simulink model "main_gilbert_R2022b"  (R2022b)
settings: Solver=VariableStepAuto  StartTime=0.0  StopTime=1  FixedStep=0.01  RelTol=1e-3
libraries: dspsigops x3, commchan3 x2, simulink x2, commsink2 x2, dspvision x2, commblkcod2 x2, commdigbbndpm3 x2, commfilt2 x2, dspstat3 x1, commrandsrc3 x1
settings Model: Creator=avyamalhotra  LastModifiedBy=Tenna Yuan

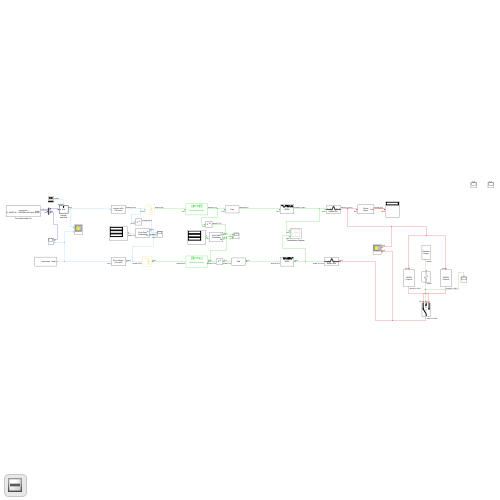
[thumbnail: Simulink's stored preview of the top-level diagram]
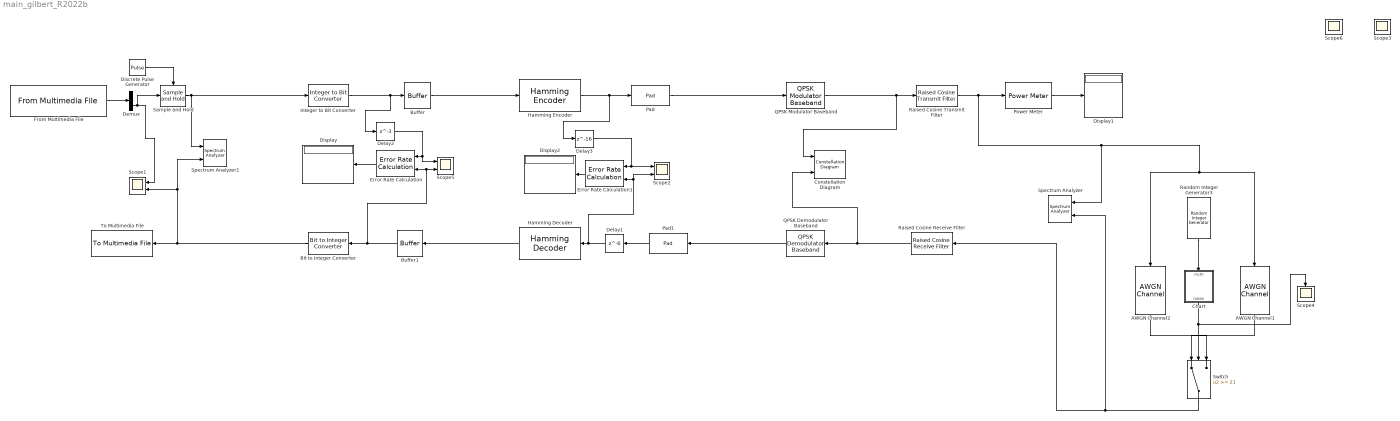
== system main_gilbert_R2022b ==
  AWGN Channel1 : commchan3/AWGN Channel  InputProcessing=Columns as channels (frame based)  noiseMode="Signal to noise ratio  (SNR)"  EbNodB=2  EsNodB=10  SNRdB=21  bitsPerSym=4  Ps=1  Tsym=(9.765625e-08 * 1)  variance=1  seed=67
  AWGN Channel2 : commchan3/AWGN Channel  InputProcessing=Columns as channels (frame based)  noiseMode="Signal to noise ratio  (SNR)"  EbNodB=2  EsNodB=10  SNRdB=9  bitsPerSym=4  Ps=1  Tsym=(9.765625e-08 * 1)  variance=1  seed=67
  Bit to Integer Converter : simulink/Logic and Bit Operations/Bit to Integer Converter  nbits=32  bitOrder=MSB first  signedOutputValues=Signed  outDtype=Inherit via internal rule  outDtypeSigned=int16
  Buffer : Buffer  N=4  OutputFrames=off
  Buffer1 : Buffer  N=32  OutputFrames=off
  Chart : Stateflow chart  TreatAsAtomicUnit=on
  Constellation Diagram : ConstellationDiagram  NumInputPorts=2  WindowPosition=[382.000000,84.000000,600.000000,600.000000,]  ScopeFrameLocation=window  SamplesPerSymbol=100  SymbolsToDisplaySource=Property  SymbolsToDisplay=200  ReferenceConstellation="{[0.70711+0.70711i        -0.70711+0.70711i        -0.70711-0.70711i         0.70711-0.70711i][0.7071+0.7071i          -0.7071+0.7071i          -0.7071-0.7071i            0.707-0.7071i]}"  XLimits=[-1.46,1.46]  YLimits=[-1.38,1.38]  ShowLegend=on
  Delay1 : Delay  DelayLength=6  InitialCondition=0
  Delay2 : Delay  DelayLength=3  InitialCondition=0
  Delay3 : Delay  DelayLength=16  InitialCondition=0
  Demux : Demux  Outputs=2
  Discrete Pulse Generator : DiscretePulseGenerator  SampleTime=1/40000
  Display : Display
  Display1 : Display
  Display2 : Display
  Error Rate Calculation : commsink2/Error Rate Calculation  N=0  st_delay=0  cp_mode=Entire frame  subframe=[]  PMode=Port  WsName=ErrorVec  RsMode2=off  stop=off  numErr=100  maxBits=1e6
  Error Rate Calculation1 : commsink2/Error Rate Calculation  N=0  st_delay=0  cp_mode=Entire frame  subframe=[]  PMode=Port  WsName=ErrorVec  RsMode2=off  stop=off  numErr=100  maxBits=1e6
  From Multimedia File : dspvision/From Multimedia File  inputFilename=D:\Documents\Uni\Year_3\Academics\ELEC_391\ELEC391-Communications-Systems\Simulink component\sound.wav  readRange=[1 Inf]  loop=on  numPlays=1  outputStreams=Audio only  videoDataType=single  audioDataType=int16  inheritSampleTime=on  userDefinedSampleTime=1/30  noAudioOutput=off  isIntensityVideo=off  fourcc=RGB  colorVideoFormat=Separate color signals  outputEOF=off  dataOrg=Column-major  audioFrameSize=1  computeAudioFrameSize=off  outSamplingMode=Sample based
      settings: LibrarySourceBlock=dspsrcs4/From Multimedia File
  Hamming Decoder : commblkcod2/Hamming Decoder  n=7  k=4
  Hamming Encoder : commblkcod2/Hamming Encoder  n=7  k=4
  Integer to Bit Converter : simulink/Logic and Bit Operations/Integer to Bit Converter  nbits=32  signedInputValues=Signed  bitOrder=MSB first  outDtype=double
  Pad : dspsigops/Pad  padAlong=Columns  dimsToPad=1  valSrc=Specify via dialog  padVal=0  spec=Output size  padNumOutRowsSpecMethod=User-specified  numOutRows=8  padNumOutColsSpecMethod=User-specified  numOutCols=7  isVarDimsMode=off  padBeginning=0  padEnd=0  outSizeMode=User-specified  outSize=1  padSigAt=End  trunc_flag=None  roundingMode=Floor  overflowMode=off  truncOrWrapMode=Truncate  wrap_flag=None
  Pad1 : dspsigops/Pad  padAlong=Columns  dimsToPad=1  valSrc=Specify via dialog  padVal=0  spec=Output size  padNumOutRowsSpecMethod=User-specified  numOutRows=7  padNumOutColsSpecMethod=User-specified  numOutCols=1  isVarDimsMode=off  padBeginning=0  padEnd=0  outSizeMode=User-specified  outSize=1  padSigAt=End  trunc_flag=None  roundingMode=Floor  overflowMode=off  truncOrWrapMode=Truncate  wrap_flag=None
  Power Meter : dspstat3/Power Meter  Measurement=Average power  ReferenceLoad=1  OutputPowerUnits=Watts  WindowLength=256  OverlapLength=255  AllowArbitraryInputLength=on  ComputeCCDF=off  PowerRange=50  PowerResolution=0.1  CCDFOutput=Relative power (dB above average power)  ProbabilityVector=[ 10; 1; 0.1; 0.01; 0.001; 0.0001 ]  RelativePowerVector=[ 0; 3; 6; 9; 12 ]  ResetPort=off  SimulateUsing=Code generation
      settings: LibrarySourceBlock=commutil2/Power Meter
  QPSK Demodulator Baseband : commdigbbndpm3/QPSK Demodulator Baseband  OutType=Bit  DecType=Hard decision  VarSource=Dialog  Variance=1  Dec=Gray  Ph=pi/4  outDtype1=Inherit via internal rule  outDtype2=Inherit via internal rule  derotateFactorWordLen=16  derotateFactorDataTypeStr=Inherit: Same word length as input  derotateFactorLastDataTypeStr=Inherit: Same word length as input
  QPSK Modulator Baseband : commdigbbndpm3/QPSK Modulator Baseband  InType=Bit  Enc=Gray  Ph=pi/4  outDtype=double  outWordLen=16  outUDDataType=sfix(16)  outFracLenMode=Best precision  outFracLen=15  outDataTypeStr=double  outLastDataTypeStr=double
  Raised Cosine Receive Filter : commfilt2/Raised Cosine Receive Filter  filtType=Square root  R=0.001  filtSpan=10  N=8  downFactor=8  downOffset=0  filterGain=1  RateOptions=Allow multirate processing  framing=Mute  checkCoeff=off  variableName=rcRxFilt  currentFiltSpan=10  D=5  inputOffset=0  sampMode=Mute  saveAsFlag=0  rateMode=Downsampling  checkGain=Normalized  launchFVT=on  roundingMode=Ceiling  overflowMode=off  coeffDataTypeStr=Inherit: Same word length as input  coeffMin=[]  coeffMax=[]  coeffLastDataTypeStr=Inherit: Same word length as input  accumDataTypeStr=Inherit: Same as product output  accumLastDataTypeStr=Inherit: Same as product output  outputDataTypeStr=Inherit: Same as accumulator  outputMin=[]  outputMax=[]  outputLastDataTypeStr=Inherit: Same as accumulator
  Raised Cosine Transmit Filter : commfilt2/Raised Cosine Transmit Filter  filtType=Square root  R=0.001  filtSpan=10  N=8  filterGain=1  RateOptions=Allow multirate processing  framing=Mute  checkCoeff=off  variableName=rcTxFilt  checkGain=Normalized  sampMode=Mute  saveAsFlag=0  currentFiltSpan=10  D=(10)/2  launchFVT=on  roundingMode=Floor  overflowMode=off  coeffDataTypeStr=Inherit: Same word length as input  coeffMin=[]  coeffMax=[]  coeffLastDataTypeStr=Inherit: Same word length as input  outputDataTypeStr=Inherit: Same as accumulator  outputMin=[]  outputMax=[]  outputLastDataTypeStr=Inherit: Same as accumulator
  Random Integer Generator3 : commrandsrc3/Random Integer Generator  SetSize=101  SeedSource=Parameter  Seed=9  SampleTime=1e-4  SamplesPerFrame=1  OutputDataType=double  SimulateUsing=Interpreted execution
  Sample and Hold : dspsigops/Sample and Hold  trig=Rising edge  initCond=0  latchinput=off
  Scope1 : Scope  NumInputPorts=2
  Scope2 : Scope  NumInputPorts=2
  Scope3 : Scope
  Scope4 : Scope
  Scope5 : Scope  NumInputPorts=2
  Scope6 : Scope
  Spectrum Analyzer : SpectrumAnalyzer  NumInputPorts=2  DefaultConfigurationName=spbscopes.SpectrumAnalyzerBlockCfg
  Spectrum Analyzer1 : SpectrumAnalyzer  NumInputPorts=2  DefaultConfigurationName=spbscopes.SpectrumAnalyzerBlockCfg
  Switch : Switch  Threshold=21  SaturateOnIntegerOverflow=off  InputSameDT=off
  To Multimedia File : dspvision/To Multimedia File  outputFilename=C:\Downloads\output.wav  streamSelection=Audio only  videoCompressor=None (uncompressed)  audioCompressor=None (uncompressed)  imagePorts=Separate color signals  fileType=WAV  audioDatatype=16-bit integer  fourcc=RGB  videoQuality=75  mj2000CompFactor=10
      settings: LibrarySourceBlock=dspsnks4/To Multimedia File
  wires:
  From Multimedia File/1 -> Demux/1
  Discrete Pulse Generator/1 -> Sample and Hold/Trigger
  Integer to Bit Converter/1 -> Delay2/1, Buffer/1
  Buffer/1 -> Hamming Encoder/1
  Sample and Hold/1 -> Integer to Bit Converter/1, Spectrum Analyzer1/1
  Hamming Decoder/1 -> Buffer1/1
  Demux/2 -> Sample and Hold/1, Scope1/1
  Hamming Encoder/1 -> Delay3/1, Pad/1
  Error Rate Calculation/1 -> Display/1
  Power Meter/1 -> Display1/1
  Pad1/1 -> Delay1/1
  Buffer1/1 -> Scope5/2, Error Rate Calculation/2, Bit to Integer Converter/1
  Delay1/1 -> Hamming Decoder/1, Scope2/2, Error Rate Calculation1/2
  Switch/1 -> Spectrum Analyzer/2, Raised Cosine Receive Filter/1
  Error Rate Calculation1/1 -> Display2/1
  Delay3/1 -> Error Rate Calculation1/1, Scope2/1
  Bit to Integer Converter/1 -> Scope1/2, Spectrum Analyzer1/2, To Multimedia File/1
  Delay2/1 -> Scope5/1, Error Rate Calculation/1
  Raised Cosine Receive Filter/1 -> Constellation Diagram/2, QPSK Demodulator Baseband/1
  QPSK Demodulator Baseband/1 -> Pad1/1
  QPSK Modulator Baseband/1 -> Constellation Diagram/1, Raised Cosine Transmit Filter/1
  Pad/1 -> QPSK Modulator Baseband/1
  AWGN Channel2/1 -> Switch/3
  AWGN Channel1/1 -> Switch/1
  Raised Cosine Transmit Filter/1 -> Spectrum Analyzer/1, AWGN Channel2/1, AWGN Channel1/1, Power Meter/1
  Random Integer Generator3/1 -> Chart/1(num)
  Chart/1(noise) -> Scope4/1, Switch/2

== stateflow chart main_gilbert_R2022b/Chart ==
  state Good_state
    noise=21;
  state Bad_state
    noise=9;
  (default) -> Good_state
  Bad_state -> Bad_state [order 2] : [num<=75]
  Good_state -> Bad_state [order 1] : [num<=3]
  Good_state -> Good_state [order 2] : [num<=97]
  Bad_state -> Good_state [order 1] : [num<=25]
  data: noise output; num input
